simulink model "mavsim_chap3"  (R2021b)
settings: Solver=ode45  StartTime=0.0  StopTime=10000  RelTol=1e-3  EnableMultiTasking=on
InitFcn:
  | addpath('../chap2')
  | addpath('../parameters/')
  | aerosonde_parameters
model workspace (MATLAB code in the model file):
  | aerosonde_parameters
undefined symbols (not defined in the file or in its folder): drawAircraft, plotMAVStateVariables
libraries: simulink x6
settings Model: Creator=beard  LastModifiedBy=zhour
settings SolverCC: AlgebraicLoopSolver=TrustRegion
settings DataIOCC: LimitDataPoints=on  SaveFormat=Array  SignalLoggingSaveFormat=ModelDataLogs  ReturnWorkspaceOutputs=off
settings OptimizationCC: ExpressionDepthLimit=2147483647  InitFltsAndDblsToZero=on  LifeSpan=inf
settings DebuggingCC: UnderspecifiedInitializationDetection=Classic  MergeDetectMultiDrivingBlocksExec=none  SolverPrmCheckMsg=warning  FcnCallInpInsideContextMsg=warning  AllowSymbolicDim=off  StateNameClashWarn=warning  SFUnexpectedBacktrackingDiag=warning  SFNoUnconditionalDefaultTransitionDiag=warning  SFExecutionAtInitializationDiag=none  SFMachineParentedDataDiag=warning  ArithmeticOperatorsInVariantConditions=warning
settings HardwareCC: ProdBitPerPointer=32  ProdBitPerSizeT=32  ProdBitPerPtrDiffT=32  ProdLargestAtomicFloat=None  ProdIntDivRoundTo=Undefined  ProdEndianess=Unspecified  ProdWordSize=32  ProdHWDeviceType=32-bit Generic
settings ModelReferenceCC: PropagateSignalLabelsOutOfModel=off
settings SFSimCC: SimUseLocalCustomCode=off  CustomCodeUndefinedFunction=UseInterfaceOnly
settings RTWCC: RTWUseLocalCustomCode=off
settings CodeAppCC: StateflowObjectComments=on
settings GRTTargetCC: TargetLangStandard=C89/C90 (ANSI)  CombineOutputUpdateFcns=off  GRTInterface=on
settings ConfigComp: CovMetricSettings=dw  CovSaveCumulativeToWorkspaceVar=on  CovSaveSingleToWorkspaceVar=on  CovExternalEMLEnable=off  CovSFcnEnable=off

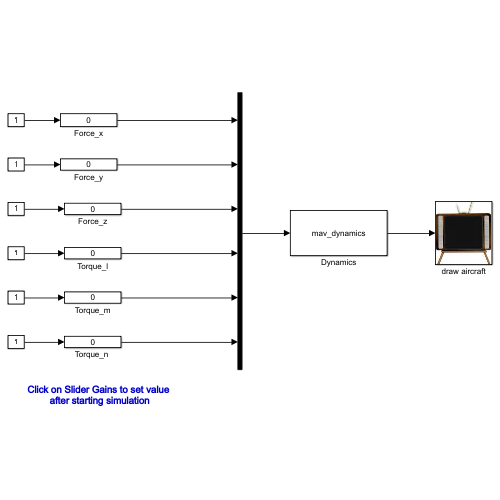
[thumbnail: Simulink's stored preview of the top-level diagram]
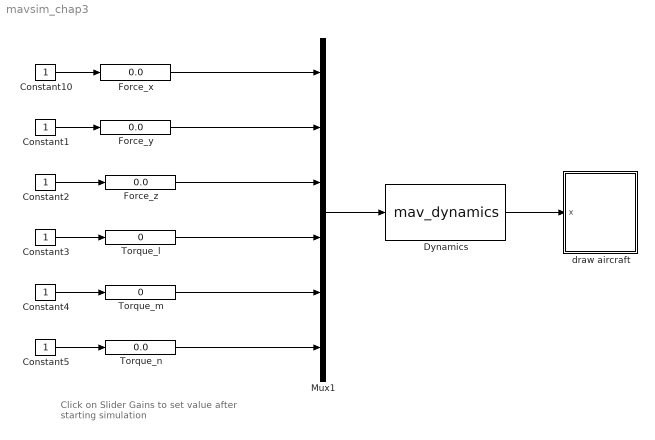
== system mavsim_chap3 ==
  note: Click on Slider Gains to set value
      | after starting simulation
  Constant{1..5,10} (6 alike) : Constant
  Dynamics : S-Function  InitFcn=|  FunctionName=mav_dynamics  Parameters=MAV  SFunctionDeploymentMode=off  EnableBusSupport=off
      | % G = Jx*Jz - Jxz^2;
      | % g1 = Jxz*(Jx - Jy + Jz)/G;
      | % g2 = (Jz*(Jz - Jy) + Jxz^2)/G;
      | % g3 = Jz/G;
      | % g4 = Jxz/G;
      | % g5 = (Jz - Jx)/Jy;
      | % g6 = Jxz/Jy;
      | % g7 = ((Jx - Jy)*Jx + Jxz^2)/G;
      | % g8 = Jx/G;
      | % 
      | % MAV.pn0 = 0;
      | % MAV.pe0 = 0;
      | % MAV.pd0 = 0;
      | % MAV.u0 = 0;
      | % MAV.v0 = 0;
      | % MAV.w0 = 0;
      | % MAV.e0 = 0;
      | % MAV.e1 = 0;
      | % MAV.e2 = 0;
      | % MAV.p0 = 0;
      | % MAV.q0 = 0;
      | % MAV.r0 = 0;
  Force_x : simulink/Math Operations/Slider Gain  gain=0.0  low=-1  high=1
  Force_y : simulink/Math Operations/Slider Gain  gain=0.0  low=-1  high=1
  Force_z : simulink/Math Operations/Slider Gain  gain=0.0  low=-1  high=1
  Mux1 : Mux  Inputs=6
  Torque_l : simulink/Math Operations/Slider Gain  gain=0  low=-0.1  high=0.1
  Torque_m : simulink/Math Operations/Slider Gain  gain=0  low=-0.1  high=0.1
  "Torque_n " : simulink/Math Operations/Slider Gain  gain=0.0  low=-0.1  high=0.1
  draw aircraft : Subsystem
      mask Display: image(imread('../chap2/tv.jpg'))
  wires:
  Constant5/1 -> "Torque_n "/1
  Constant10/1 -> Force_x/1
  Constant1/1 -> Force_y/1
  Constant2/1 -> Force_z/1
  Dynamics/1 -> draw aircraft/1(x)
  Force_z/1 -> Mux1/3
  Force_y/1 -> Mux1/2
  Force_x/1 -> Mux1/1
  "Torque_n "/1 -> Mux1/6
  Constant4/1 -> Torque_m/1
  Torque_m/1 -> Mux1/5
  Constant3/1 -> Torque_l/1
  Torque_l/1 -> Mux1/4
  Mux1/1 -> Dynamics/1

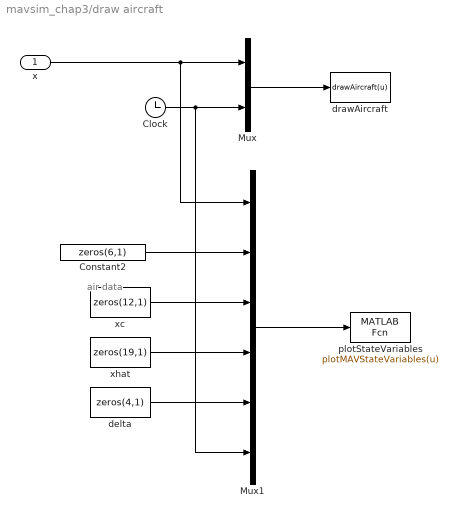
== system mavsim_chap3/draw aircraft ==
  note: air data
  x : Inport
  Clock : Clock
  Constant2 : Constant  Value=zeros(6,1)
  Mux : Mux  Inputs=2
  Mux1 : Mux  Inputs=6
  delta : Constant  Value=zeros(4,1)
  drawAircraft : MATLABFcn  MATLABFcn=drawAircraft(u)  OutputDimensions=0  SampleTime=0.1
  plotStateVariables : MATLABFcn  MATLABFcn=plotMAVStateVariables(u)  OutputDimensions=0  SampleTime=0.1
  xc : Constant  Value=zeros(12,1)
  xhat : Constant  Value=zeros(19,1)
  wires:
  Mux/1 -> drawAircraft/1
  x/1 -> Mux/1, Mux1/1
  Clock/1 -> Mux/2, Mux1/6
  Mux1/1 -> plotStateVariables/1
  xhat/1 -> Mux1/4
  xc/1 -> Mux1/3
  delta/1 -> Mux1/5
  Constant2/1 -> Mux1/2
